simulink model "AUTOCS1"  (R2024a)
settings: Solver=VariableStepAuto  StartTime=0.0  StopTime=765  RelTol=1e-3
undefined symbols (not defined in the file): canChannel, Ion, Lithium
libraries: canlib x5, canmsglib x4, svdutilitieslib x2, dspnetwork x2, simulink x1, spsBatteryLib x1, spsDCMachineLib x1, autolibshared x1, sps_lib x1
settings Model: Creator=Manikanta  LastModifiedBy=Manikanta
settings DebuggingCC: SigSpecEnsureSampleTimeMsg=none

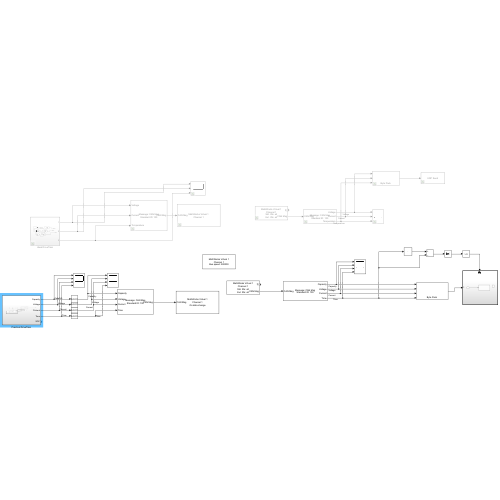
[thumbnail: Simulink's stored preview of the top-level diagram]
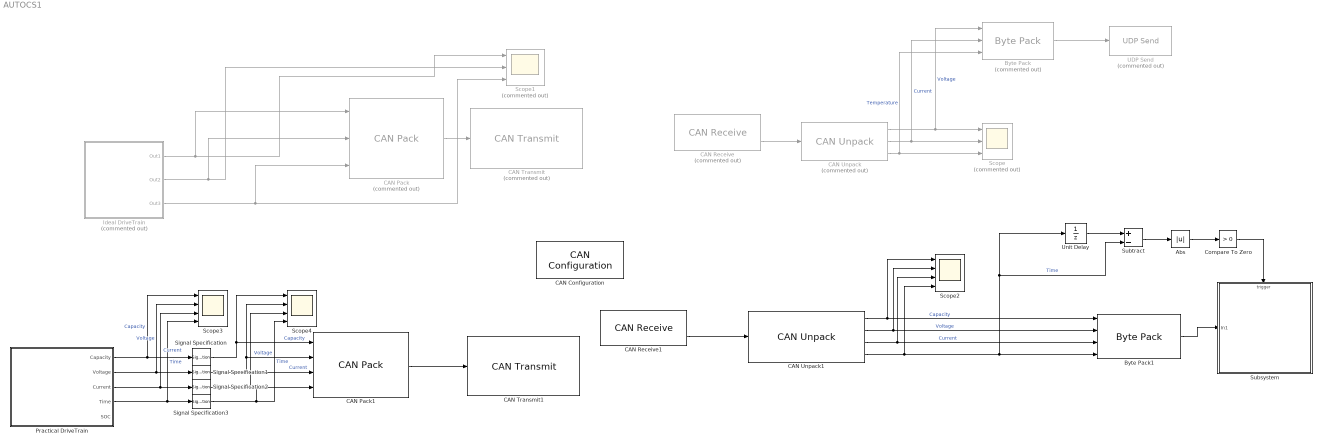
== system AUTOCS1 ==
  Abs : Abs  ZeroCross=off  SaturateOnIntegerOverflow=off
  Byte Pack : svdutilitieslib/Byte Pack  Commented=on  maskPackedDataType=uint8  datatypes={'single','single','single'}  byteAlign=1  blockPlatform=arduinoert
      settings: LibrarySourceBlock=mcblib/Signal Management/Byte Pack
  Byte Pack1 : svdutilitieslib/Byte Pack  maskPackedDataType=uint8  datatypes={'single','single','single','single'}  byteAlign=1  blockPlatform=arduinoert
      settings: LibrarySourceBlock=mcblib/Signal Management/Byte Pack
  CAN Configuration : canlib/CAN Configuration  BlockHandle=290.0002  Device=MathWorks Virtual 1 (Channel 1)  DeviceMenu=MathWorks Virtual 1 (Channel 1)  ObjConstructor=canChannel('MathWorks', 'Virtual 1', 1)  BusSpeed=500000  EnableBitParameters=off  AckMode=Normal
  CAN Pack : canmsglib/CAN Pack  Commented=on  MsgList=(none)  MsgName=CAN Msg  MsgIDType=Standard (11-bit identifier)  MsgIdentifier=100  MsgLength=8  Remote=off  ApplyMinMax=off  BusOutput=off  SignalInfo={ 'Voltage', '0', '16', 'LE', 'signed', 'Standard', '0', '1', '0', '-Inf', 'Inf'; 'Current', '16', '16', 'LE', 'signed', 'Standard', '0', '1', '0', '-Inf', 'Inf'; 'Temperature', '32', '16', 'LE', 'signed', 'Standard', '0', '1', '0', '-Inf', 'Inf' }
      settings: LibrarySourceBlock=canlib/CAN Pack  DataFormat=manually specified signals
  CAN Pack1 : canmsglib/CAN Pack  MsgList=(none)  MsgName=CAN Msg  MsgIDType=Standard (11-bit identifier)  MsgIdentifier=100  MsgLength=8  Remote=off  ApplyMinMax=off  BusOutput=off  SignalInfo={ 'Capacity', '0', '16', 'LE', 'signed', 'Standard', '0', '0.01', '0', '-Inf', 'Inf'; 'Voltage', '16', '16', 'LE', 'signed', 'Standard', '0', '0.01', '0', '-Inf', 'Inf'; 'Current', '32', '16', 'LE', 'signed', 'Standard', '0', '0.01', '0', '-Inf', 'Inf'; 'Time', '48', '16', 'LE', 'signed', 'Standard', '0', '1', '0', '-Inf', 'Inf' }
      settings: LibrarySourceBlock=canlib/CAN Pack  DataFormat=manually specified signals
  CAN Receive : canlib/CAN Receive  Commented=on  BlockHandle=302.0002  Device=MathWorks Virtual 1 (Channel 1)  DeviceMenu=MathWorks Virtual 1 (Channel 1)  ObjConstructor=canChannel('MathWorks', 'Virtual 1', 1)  EnableStandardIDsFilter=off  StdIDsCombo=Allow all  StandardIDs=0  EnableExtendedIDsFilter=off  ExtIDsCombo=Allow all  ExtendedIDs=0  SampleTime=1  MsgsPerTimestep=all  InternalFilterUpdateStatus=on  BusOutput=off
  CAN Receive1 : canlib/CAN Receive  BlockHandle=305.0002  Device=MathWorks Virtual 1 (Channel 1)  DeviceMenu=MathWorks Virtual 1 (Channel 1)  ObjConstructor=canChannel('MathWorks', 'Virtual 1', 1)  EnableStandardIDsFilter=off  StdIDsCombo=Allow all  StandardIDs=0  EnableExtendedIDsFilter=off  ExtIDsCombo=Allow all  ExtendedIDs=0  SampleTime=0.01  MsgsPerTimestep=1  InternalFilterUpdateStatus=on  BusOutput=off
  CAN Transmit : canlib/CAN Transmit  Commented=on  BlockHandle=308.0002  Device=MathWorks Virtual 1 (Channel 1)  DeviceMenu=MathWorks Virtual 1 (Channel 1)  ObjConstructor=canChannel('MathWorks', 'Virtual 1', 1)  EnableEventTransmit=off  EnablePeriodicTransmit=off  MessagePeriod=1.000
  CAN Transmit1 : canlib/CAN Transmit  BlockHandle=310.0002  Device=MathWorks Virtual 1 (Channel 1)  DeviceMenu=MathWorks Virtual 1 (Channel 1)  ObjConstructor=canChannel('MathWorks', 'Virtual 1', 1)  EnableEventTransmit=on  EnablePeriodicTransmit=off  MessagePeriod=0.025
  CAN Unpack : canmsglib/CAN Unpack  Commented=on  MsgList=(none)  MsgName=CAN Msg  MsgIDType=Standard (11-bit identifier)  MsgIdentifier=100  MsgLength=8  SignalInfo={ 'Voltage', '0', '16', 'LE', 'signed', 'Standard', '0', '1', '.01', '-Inf', 'Inf'; 'Current', '16', '16', 'LE', 'signed', 'Standard', '0', '1', '0.01', '-Inf', 'Inf'; 'Temperature', '32', '16', 'LE', 'signed', 'Standard', '0', '1', '0.01', '-Inf', 'Inf' }  IDPort=off  TimestampPort=off  ErrorPort=off  RemotePort=off  LengthPort=off  StatusPort=off  ApplyMinMax=off
      settings: LibrarySourceBlock=canlib/CAN Unpack
  CAN Unpack1 : canmsglib/CAN Unpack  MsgList=(none)  MsgName=CAN Msg  MsgIDType=Standard (11-bit identifier)  MsgIdentifier=100  MsgLength=8  SignalInfo={ 'Capacity', '0', '16', 'LE', 'signed', 'Standard', '0', '.01', '0', '-Inf', 'Inf'; 'Voltage', '16', '16', 'LE', 'signed', 'Standard', '0', '.01', '0', '-Inf', 'Inf'; 'Current', '32', '16', 'LE', 'signed', 'Standard', '0', '.01', '0', '-Inf', 'Inf'; 'Time', '48', '16', 'LE', 'signed', 'Standard', '0', '1', '0', '-Inf', 'Inf' }  IDPort=off  TimestampPort=off  ErrorPort=off  RemotePort=off  LengthPort=off  StatusPort=off  ApplyMinMax=off
      settings: LibrarySourceBlock=canlib/CAN Unpack
  Compare To Zero : simulink/Logic and Bit Operations/Compare To Zero  relop=>  OutDataTypeStr=boolean  ZeroCross=off
  Ideal DriveTrain : Subsystem  Commented=on
  Practical DriveTrain : Subsystem
  Scope : Scope  Commented=on  NumInputPorts=3
  Scope1 : Scope  Commented=on  NumInputPorts=3
  Scope2 : Scope  NumInputPorts=4
  Scope3 : Scope  NumInputPorts=4
  Scope4 : Scope  NumInputPorts=4
  Signal Specification{,1..3} (4 alike) : SignalSpecification  SampleTime=0.01
  Subsystem : Subsystem
  Subtract : Sum  Inputs=+-
  UDP Send : dspnetwork/UDP Send  Commented=on  remoteURL='127.0.0.1'  remotePort=7005  localURL='0.0.0.0'  localPortSource=Automatically determine  localPort=-1  sendBufferSize=8192  sampletime=-1  blockPlatform=[]  separateLengthPort=0
      settings: LibrarySourceBlock=dspsnks4/UDP Send
  Unit Delay : UnitDelay  SampleTime=-1  HasFrameUpgradeWarning=on
  wires:
  CAN Pack/1 -> CAN Transmit/1
  CAN Receive/2 -> CAN Unpack/1
  CAN Unpack/1 -> Scope/1, Byte Pack/1  "Voltage"
  CAN Unpack/2 -> Byte Pack/2, Scope/2  "Current"
  CAN Unpack/3 -> Byte Pack/3, Scope/3  "Temperature"
  Ideal DriveTrain/1(Out1) -> CAN Pack/1, Scope1/1
  Ideal DriveTrain/3(Out3) -> CAN Pack/3, Scope1/3
  Ideal DriveTrain/2(Out2) -> CAN Pack/2, Scope1/2
  Byte Pack/1 -> UDP Send/1
  CAN Pack1/1 -> CAN Transmit1/1
  CAN Receive1/2 -> CAN Unpack1/1
  CAN Unpack1/1 -> Scope2/1, Byte Pack1/1  "Capacity"
  CAN Unpack1/2 -> Scope2/2, Byte Pack1/2  "Voltage"
  CAN Unpack1/3 -> Scope2/3, Byte Pack1/3  "Current"
  CAN Unpack1/4 -> Subtract/2, Unit Delay/1, Byte Pack1/4, Scope2/4  "Time"
  Practical DriveTrain/4(Time) -> Scope3/4, Signal Specification3/1  "Time"
  Practical DriveTrain/3(Current) -> Scope3/3, Signal Specification2/1  "Current"
  Practical DriveTrain/2(Voltage) -> Scope3/2, Signal Specification1/1  "Voltage"
  Practical DriveTrain/1(Capacity) -> Scope3/1, Signal Specification/1  "Capacity"
  Signal Specification/1 -> Scope4/1, CAN Pack1/1  "Capacity"
  Signal Specification1/1 -> Scope4/2, CAN Pack1/2  "Voltage"
  Signal Specification2/1 -> Scope4/3, CAN Pack1/3  "Current"
  Signal Specification3/1 -> Scope4/4, CAN Pack1/4  "Time"
  Byte Pack1/1 -> Subsystem/1(In1)
  Unit Delay/1 -> Subtract/1
  Subtract/1 -> Abs/1
  Compare To Zero/1 -> Subsystem/Trigger
  Abs/1 -> Compare To Zero/1

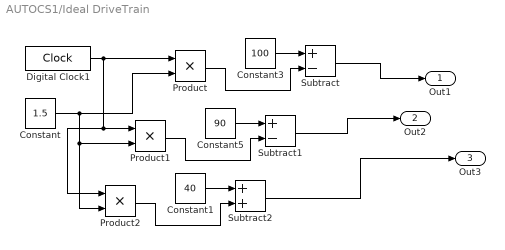
== system AUTOCS1/Ideal DriveTrain ==
  Constant : Constant  Value=1.5
  Constant1 : Constant  Value=40
  Constant3 : Constant  Value=100
  Constant5 : Constant  Value=90
  Digital Clock1 : DigitalClock  SampleTime=.001
  Product : Product
  Product1 : Product
  Product2 : Product
  Subtract : Sum  Inputs=+-
  Subtract1 : Sum  Inputs=+-
  Subtract2 : Sum
  Out1 : Outport
  Out2 : Outport  Port=2
  Out3 : Outport  Port=3
  wires:
  Constant3/1 -> Subtract/1
  Constant/1 -> Product2/2, Product1/2, Product/2
  Digital Clock1/1 -> Product2/1, Product1/1, Product/1
  Product2/1 -> Subtract2/2
  Constant1/1 -> Subtract2/1
  Product1/1 -> Subtract1/2
  Constant5/1 -> Subtract1/1
  Subtract2/1 -> Out3/1
  Product/1 -> Subtract/2
  Subtract1/1 -> Out2/1
  Subtract/1 -> Out1/1

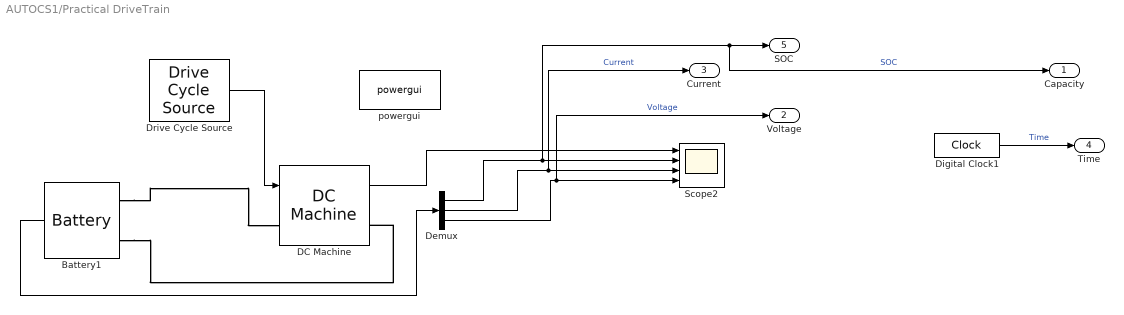
== system AUTOCS1/Practical DriveTrain ==
  Battery1 : spsBatteryLib/Battery  BatType=Lithium-Ion  ShowTempParam=off  ThermalPreset=no  ShowAgeParam=off  NomV=3.7  NomQ=2  SOC=100  Batt_Tr=30  PresetModel=on  MaxQ=2  MinV=2.775  FullV=4.3068  Dis_rate=0.86957  R=0.0185  Normal_OP=1.8087  expZone="[3.9974    0.098261]"  current=[6.5 13 32.5]  Units=Time  Tci=20  NomT=20  T2=-30  MaxQ2=4.8  FullV2=7.1  Normal_OP2=5.655  expZone2="[6.58           1]"  Rca=0.6  ti=2000  Dp=0  Neq0=0  Tsim=1e6  Ta1=25  Qeol=5.4*0.9  Reol=0.013333*1.2  Char_age=[2.3478, 3]  Dis_age=[2.3478, 10]  N1=1500  N2=10500  N3=1000  N4=1400  Ta2=45  N5=950
  DC Machine : spsDCMachineLib/DC Machine  PresetModel=No  MechanicalLoad=Torque TL  FieldType=Permanent magnet  ShowDetailedParameters=on  MeasurementBus=off  RLa="[ 3.1  0.012]"  RLf="[ 240  120]"  Laf=1.8  MachineConstant=Torque constant (N.m/A)  Ke=1.8  Kt=2  J=0.12  Bm=0  Tf=0  w0=1  Ifinit=1  TsPowergui=0  TsBlock=-1
  Demux : Demux  Outputs=3
  Digital Clock1 : DigitalClock  SampleTime=0.01
  Drive Cycle Source : autolibshared/Drive Cycle Source  cycleVar=HWFET  fileVar=cycleFTP75.mat  tfinal="765  seconds"  cycleRepeat=off  outAccPort=off  outGearPort=off  gearList=No gear data  t_wot1=5  xdot_woto=0  xdot_wot1=30  t_wot2=20  xdot_wot2=0  t_wotend=30  srcUnit=m/s  outUnit=m/s  srcAccUnit=m/s/s  outAccUnit=m/s^2  dt=0  aMode=1  faultOption=off  velBnd=2  velBndUnit=mph  inUnit=m/s  timeBnd=1  failOption=off  stopSim=off  maxFaultCnt=10  maxFaultTime=2  maxTotFaultTime=15  traceOption=off  dtTrace=1  traceWindow=10  lastDCname=FTP72  lastOutUnit=mph  lastDT=0  lastTB=1  lastSB=2  forceCalcBound=off
  Scope2 : Scope  NumInputPorts=4
  powergui : sps_lib/powergui  Priority=1  SimulationMode=Continuous  SampleTime=50e-6  frequency=60  Iterations=50  frequencyindice=0  Pbase=100e6  ErrMax=1e-4  UnitsV=kV  UnitsW=MW  buscounter=0  FunctionMessages=off  echomessages=off  EnableUseOfTLC=off  CurrentSourceSwitches=off  DisableSnubberDevices=off  DisableRonSwitches=off  DisableVfSwitches=off  DisplayEquations=off  AutomaticDiscreteSolvers=off  SolverType=Tustin/Backward Euler (TBE)  Interpol=off  ExternalGateDelay=off  methode=off  Ts=100  x0status=blocks  SPID=on  SwTol=0  HookPort=off  NonlinearTolerance=1e-4  nMaxIteration=100  ContinueOnMaxIteration=off  RestoreLinks=warning  ResistiveCurrentMeasurement=off  Frange=[0:2:500]  Ylog=off  Xlog=on  ShowGrid=off  save=off  variable=ZData  structure=0  ZoomFFT=off  StartTime=0.0  cycles=1  DisplayStyle=1  fundamental=60  FreqAxis=off  MaxFrequency=1000  frequencyindicesteady=1  RmsSteady=1  display=off
  Capacity : Outport
  Voltage : Outport  Port=2
  Current : Outport  Port=3
  Time : Outport  Port=4
  SOC : Outport  Port=5
  wires:
  Demux/2 -> Current/1, Scope2/3  "Current"
  DC Machine/1 -> Scope2/1
  Battery1/1 -> Demux/1
  Demux/1 -> Capacity/1, SOC/1, Scope2/2  "SOC"
  Demux/3 -> Voltage/1, Scope2/4  "Voltage"
  Digital Clock1/1 -> Time/1  "Time"
  Drive Cycle Source/1 -> DC Machine/1
  connections:
  Battery1/LConn1 -- DC Machine/LConn1
  Battery1/LConn2 -- DC Machine/RConn1

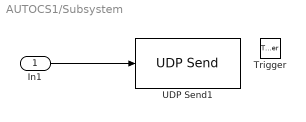
== system AUTOCS1/Subsystem ==
  In1 : Inport
  Trigger : TriggerPort  TriggerType=either  VariantControl=(inherit)  PortDimensions=1
  UDP Send1 : dspnetwork/UDP Send  remoteURL='127.0.0.1'  remotePort=7005  localURL='0.0.0.0'  localPortSource=Automatically determine  localPort=-1  sendBufferSize=8192  sampletime=-1  blockPlatform=[]  separateLengthPort=0
      settings: LibrarySourceBlock=dspsnks4/UDP Send
  wires:
  In1/1 -> UDP Send1/1
